simulink model "Simple_Kalman"  (R2020b)
settings: Solver=FixedStepAuto  StartTime=0.0  StopTime=TMax  FixedStep=DT  RelTol=1e-3
undefined symbols (not defined in the file or in its folder): CP, CP_lambda_grid, CP_theta_grid, PR_A, PR_B, PR_C, PR_L, PR_theta0, SK_A, SK_B, SK_L, SK_lambda_0, SK_R, SK_rho, SK_x0
settings Model: Creator=lpwoolcock  LastModifiedBy=lukew

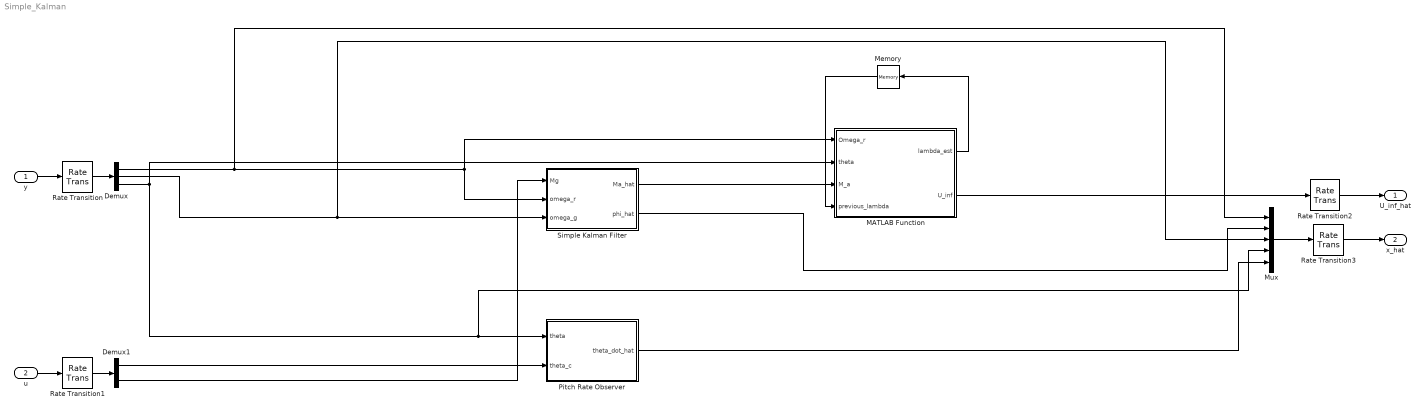
== system Simple_Kalman ==
  y : Inport  PortDimensions=[3 1]
  u : Inport  Port=2  PortDimensions=[2 1]
  Demux : Demux  Outputs=3
  Demux1 : Demux  Outputs=2
  MATLAB Function : MATLAB Function  TreatAsAtomicUnit=on
  Memory : Memory  InitialCondition=SK_lambda_0
  Mux : Mux  Inputs=5
  Pitch Rate Observer : Subsystem  TreatAsAtomicUnit=on
  Rate Transition : RateTransition  InitialCondition=zeros(3,1)  OutPortSampleTime=SK_T
  Rate Transition1 : RateTransition  InitialCondition=zeros(2,1)  OutPortSampleTime=SK_T
  Rate Transition2 : RateTransition
  Rate Transition3 : RateTransition  InitialCondition=zeros(5,1)
  Simple Kalman Filter : Subsystem  TreatAsAtomicUnit=on
  U_inf_hat : Outport  PortDimensions=1
  x_hat : Outport  Port=2  PortDimensions=[5 1]
  wires:
  Demux1/2 -> Simple Kalman Filter/1(Mg)
  Demux/1 -> Mux/1, Simple Kalman Filter/2(omega_r), MATLAB Function/1(Omega_r)
  Memory/1 -> MATLAB Function/4(previous_lambda)
  MATLAB Function/1(lambda_est) -> Memory/1
  Simple Kalman Filter/1(Ma_hat) -> MATLAB Function/3(M_a)
  MATLAB Function/2(U_inf) -> Rate Transition2/1
  Simple Kalman Filter/2(phi_hat) -> Mux/2
  Pitch Rate Observer/1(theta_dot_hat) -> Mux/5
  y/1 -> Rate Transition/1
  Demux/2 -> Mux/3, Simple Kalman Filter/3(omega_g)
  Demux/3 -> Mux/4, Pitch Rate Observer/1(theta), MATLAB Function/2(theta)
  u/1 -> Rate Transition1/1
  Demux1/1 -> Pitch Rate Observer/2(theta_c)
  Mux/1 -> Rate Transition3/1
  Rate Transition/1 -> Demux/1
  Rate Transition1/1 -> Demux1/1
  Rate Transition2/1 -> U_inf_hat/1
  Rate Transition3/1 -> x_hat/1

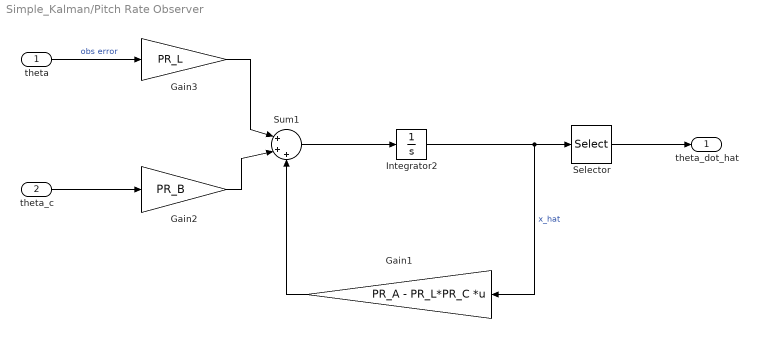
== system Simple_Kalman/Pitch Rate Observer ==
  theta : Inport
  theta_c : Inport  Port=2
  Gain1 : Gain  Gain=PR_A - PR_L*PR_C  Multiplication=Matrix(K*u)
  Gain2 : Gain  Gain=PR_B
  Gain3 : Gain  Gain=PR_L
  Integrator2 : Integrator  InitialCondition=PR_theta0
  Selector : Selector  InputPortWidth=2  IndexOptions=Index vector (dialog)  Indices=[2]  OutputSizes=1
  Sum1 : Sum  Inputs=|+++
  theta_dot_hat : Outport
  wires:
  Sum1/1 -> Integrator2/1
  Gain2/1 -> Sum1/2
  Gain3/1 -> Sum1/1
  Integrator2/1 -> Selector/1, Gain1/1  "x_hat"
  theta/1 -> Gain3/1  "obs error"
  Gain1/1 -> Sum1/3
  theta_c/1 -> Gain2/1
  Selector/1 -> theta_dot_hat/1

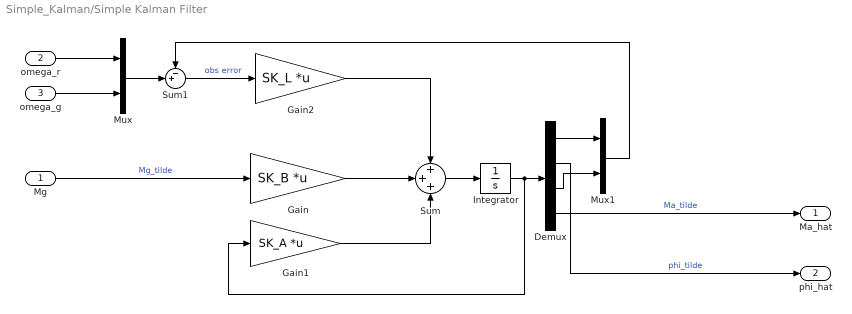
== system Simple_Kalman/Simple Kalman Filter ==
  Mg : Inport
  omega_r : Inport  Port=2
  omega_g : Inport  Port=3
  Demux : Demux
  Gain : Gain  Gain=SK_B  Multiplication=Matrix(K*u) (u vector)
  Gain1 : Gain  Gain=SK_A  Multiplication=Matrix(K*u) (u vector)
  Gain2 : Gain  Gain=SK_L  Multiplication=Matrix(K*u) (u vector)
  Integrator : Integrator  InitialCondition=SK_x0
  Mux : Mux  Inputs=2
  Mux1 : Mux  Inputs=2
  Sum : Sum  Inputs=+++
  Sum1 : Sum  Inputs=-+|
  Ma_hat : Outport
  phi_hat : Outport  Port=2
  wires:
  omega_r/1 -> Mux/1
  omega_g/1 -> Mux/2
  Mux/1 -> Sum1/2
  Sum1/1 -> Gain2/1  "obs error"
  Integrator/1 -> Gain1/1, Demux/1
  Demux/4 -> Ma_hat/1  "Ma_tilde"
  Gain/1 -> Sum/2
  Gain1/1 -> Sum/3
  Sum/1 -> Integrator/1
  Demux/3 -> Mux1/2
  Demux/1 -> Mux1/1
  Mux1/1 -> Sum1/1
  Demux/2 -> phi_hat/1  "phi_tilde"
  Mg/1 -> Gain/1  "Mg_tilde"
  Gain2/1 -> Sum/1

== matlab function Simple_Kalman/MATLAB Function ==
  data: Omega_r input; theta input; lambda_est output; M_a input; U_inf output; previous_lambda input; SK_rho parameter size=1; SK_R parameter size=1; SK_lambda_0 parameter; CP parameter; CP_theta_grid parameter; CP_lambda_grid parameter
% Computes the windspeed using a secant method with given torque
% estimation, rotor speed, and blade pitch angle
function [lambda_est, U_inf] = torque_to_windspeed(Omega_r, theta, M_a, previous_lambda, SK_rho, SK_R, SK_lambda_0, CP, CP_theta_grid, CP_lambda_grid)

    theta = max(theta, 0);

    % constant in the equation Cp/lambda^3 = C
    C = 2*M_a/(SK_rho*pi*(SK_R)^5*(Omega_r)^2);

    % Now find the root of f(lambda) = Cp/lambda^3 - C
    f = @(lambda) interp2(CP_theta_grid, CP_lambda_grid, CP, theta, lambda, 'cubic')/(lambda^3) - C;

    if isnan(f(previous_lambda))
        disp("what");
    end

    % Initial guess is previous lambda value
    [lambda_est, ~, EXITFLAG] = fzero(f, previous_lambda);

    % couldn't find valid root, just use optimal lambda for Region 2
    if EXITFLAG == -3
        lambda_est = SK_lambda_0; 
    end

    U_inf = SK_R*Omega_r/lambda_est;

end
